simulink model "VARIACION_P1_P2_P3"  (R2019b)
settings: Solver=VariableStepAuto  StartTime=0.0  StopTime=15000  RelTol=1e-3
undefined symbols (not defined in the file): n, p1, p1Aumentado, p1Disminuido, p2, p2Aumentado, p2Disminuido, p3, p3Aumentado, p3Disminuido, p6
libraries: simulink x18
settings Model: Creator=USUARIO  LastModifiedBy=USUARIO

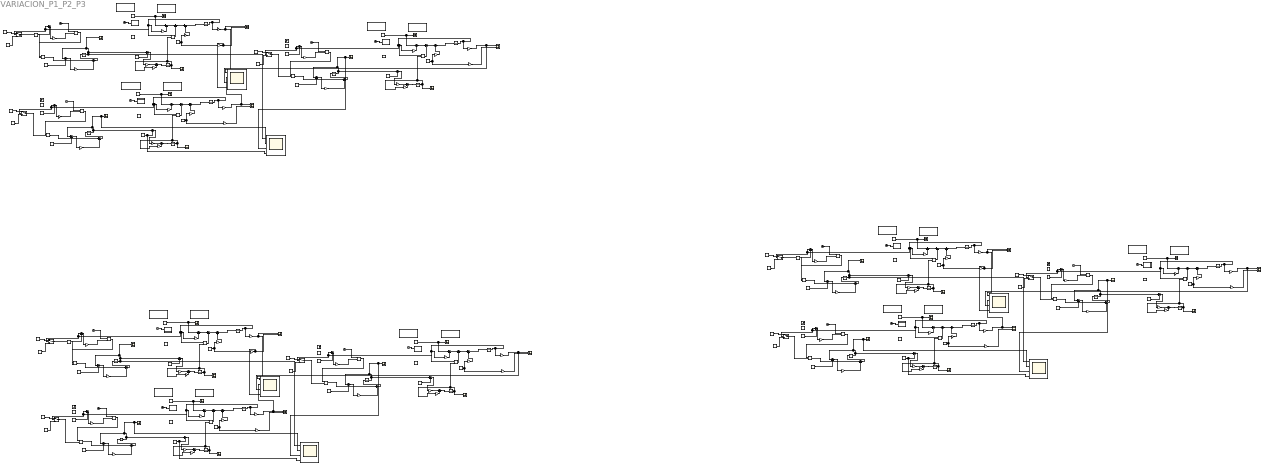
== system VARIACION_P1_P2_P3 ==
  Clock{,1..17} (18 alike) : Clock
  Constant{1..9} (9 alike) : Constant  Value=0
  Gain{1,5,11,17,19,21,23,27,32,34,37,39,41,45,50,52} (16 alike) : Gain  Gain=p1
  Gain{3..4,9..10,15..16,20,25..26,30..31,36,38,43..44,48..49,54} (18 alike) : Gain  Gain=18
  Gain{6,12,18,33,40,46,51} (7 alike) : Gain  Gain=p2
  Gain13 : Gain  Gain=p1Disminuido
  Gain{2,8,14,24,29,35,47} (7 alike) : Gain  Gain=p3
  Gain22 : Gain  Gain=p2Aumentado
  Gain28 : Gain  Gain=p2Disminuido
  Gain42 : Gain  Gain=p3Disminuido
  Gain53 : Gain  Gain=p3Aumentado
  Gain7 : Gain  Gain=p1Aumentado
  Glucosa {,1..5} (6 alike) : Constant  Value=7
  Glucosa basal{1..2,5,10..11,14,19..20,23} (9 alike) : Constant  Value=4.5
  Glucosa basal{3,6..7,12,15..16,21,24..25} (9 alike) : Constant
  Glucosa basal{4,8..9,13,17..18,22,26..27} (9 alike) : Constant  Value=0
  Grafica ingesta D{1..9} (9 alike) : Scope
  INSULINA{,1..8} (9 alike) : Scope
  Ib{,1..8} (9 alike) : Constant  Value=12
  Ingesta 75 g1 : MATLAB Function  TreatAsAtomicUnit=on
  Ingesta 75 g2 : MATLAB Function  TreatAsAtomicUnit=on
  Ingesta 75 g3 : MATLAB Function  TreatAsAtomicUnit=on
  Ingesta 75 g4 : MATLAB Function  TreatAsAtomicUnit=on
  Ingesta 75 g5 : MATLAB Function  TreatAsAtomicUnit=on
  Ingesta 75 g6 : MATLAB Function  TreatAsAtomicUnit=on
  Ingesta 75 g7 : MATLAB Function  TreatAsAtomicUnit=on
  Ingesta 75 g8 : MATLAB Function  TreatAsAtomicUnit=on
  Ingesta 75 g9 : MATLAB Function  TreatAsAtomicUnit=on
  Insulina basal{1..9} (9 alike) : Constant  Value=12
  Integrator{1,3,6,9,12,16,19,22,25} (9 alike) : Integrator  InitialCondition=7.5
  Integrator{4,7,10,13..14,17,20,23,26} (9 alike) : Integrator  InitialCondition=12
  Integrator{2,5,8,11,15,18,21,24,27} (9 alike) : Integrator
  Model Info1 : simulink/Model-Wide Utilities/Model Info  Frame=on  DisplayStringWithTags=|  HorizontalTextAlignment=Center  LeftAlignmentValue=0.5
      | Insulina constante 
      | igual a la basal
      | 
      | I(0) = Ib
  Model Info10 : simulink/Model-Wide Utilities/Model Info  Frame=on  DisplayStringWithTags=|  HorizontalTextAlignment=Center  LeftAlignmentValue=0.5
      | MODELO ORIGINAL
      | 
      | 
      | PERSONA NO DIABETICA
      | 
      | CON INSULINA VARIABLE
  Model Info11 : simulink/Model-Wide Utilities/Model Info  Frame=on  DisplayStringWithTags=|  HorizontalTextAlignment=Center  LeftAlignmentValue=0.5
      | Insulina constante 
      | igual a la basal
      | 
      | I(0) = Ib
  Model Info12 : simulink/Model-Wide Utilities/Model Info  Frame=on  DisplayStringWithTags=|  HorizontalTextAlignment=Center  LeftAlignmentValue=0.5
      | MODELO ORIGINAL
      | 
      | 
      | PERSONA NO DIABETICA
      | 
      | CON INSULINA VARIABLE
  Model Info13 : simulink/Model-Wide Utilities/Model Info  Frame=on  DisplayStringWithTags=|  HorizontalTextAlignment=Center  LeftAlignmentValue=0.5
      | Insulina constante 
      | igual a la basal
      | 
      | I(0) = Ib
  Model Info14 : simulink/Model-Wide Utilities/Model Info  Frame=on  DisplayStringWithTags=|  HorizontalTextAlignment=Center  LeftAlignmentValue=0.5
      | MODELO ORIGINAL
      | 
      | 
      | PERSONA NO DIABETICA
      | 
      | CON INSULINA VARIABLE
  Model Info15 : simulink/Model-Wide Utilities/Model Info  Frame=on  DisplayStringWithTags=|  HorizontalTextAlignment=Center  LeftAlignmentValue=0.5
      | Insulina constante 
      | igual a la basal
      | 
      | I(0) = Ib
  Model Info16 : simulink/Model-Wide Utilities/Model Info  Frame=on  DisplayStringWithTags=|  HorizontalTextAlignment=Center  LeftAlignmentValue=0.5
      | MODELO ORIGINAL
      | 
      | 
      | PERSONA NO DIABETICA
      | 
      | CON INSULINA VARIABLE
  Model Info17 : simulink/Model-Wide Utilities/Model Info  Frame=on  DisplayStringWithTags=|  HorizontalTextAlignment=Center  LeftAlignmentValue=0.5
      | Insulina constante 
      | igual a la basal
      | 
      | I(0) = Ib
  Model Info18 : simulink/Model-Wide Utilities/Model Info  Frame=on  DisplayStringWithTags=|  HorizontalTextAlignment=Center  LeftAlignmentValue=0.5
      | MODELO ORIGINAL
      | 
      | 
      | PERSONA NO DIABETICA
      | 
      | CON INSULINA VARIABLE
  Model Info2 : simulink/Model-Wide Utilities/Model Info  Frame=on  DisplayStringWithTags=|  HorizontalTextAlignment=Center  LeftAlignmentValue=0.5
      | MODELO ORIGINAL
      | 
      | 
      | PERSONA NO DIABETICA
      | 
      | CON INSULINA VARIABLE
  Model Info3 : simulink/Model-Wide Utilities/Model Info  Frame=on  DisplayStringWithTags=|  HorizontalTextAlignment=Center  LeftAlignmentValue=0.5
      | Insulina constante 
      | igual a la basal
      | 
      | I(0) = Ib
  Model Info4 : simulink/Model-Wide Utilities/Model Info  Frame=on  DisplayStringWithTags=|  HorizontalTextAlignment=Center  LeftAlignmentValue=0.5
      | MODELO ORIGINAL
      | 
      | 
      | PERSONA NO DIABETICA
      | 
      | CON INSULINA VARIABLE
  Model Info5 : simulink/Model-Wide Utilities/Model Info  Frame=on  DisplayStringWithTags=|  HorizontalTextAlignment=Center  LeftAlignmentValue=0.5
      | Insulina constante 
      | igual a la basal
      | 
      | I(0) = Ib
  Model Info6 : simulink/Model-Wide Utilities/Model Info  Frame=on  DisplayStringWithTags=|  HorizontalTextAlignment=Center  LeftAlignmentValue=0.5
      | MODELO ORIGINAL
      | 
      | 
      | PERSONA NO DIABETICA
      | 
      | CON INSULINA VARIABLE
  Model Info7 : simulink/Model-Wide Utilities/Model Info  Frame=on  DisplayStringWithTags=|  HorizontalTextAlignment=Center  LeftAlignmentValue=0.5
      | Insulina constante 
      | igual a la basal
      | 
      | I(0) = Ib
  Model Info8 : simulink/Model-Wide Utilities/Model Info  Frame=on  DisplayStringWithTags=|  HorizontalTextAlignment=Center  LeftAlignmentValue=0.5
      | MODELO ORIGINAL
      | 
      | 
      | PERSONA NO DIABETICA
      | 
      | CON INSULINA VARIABLE
  Model Info9 : simulink/Model-Wide Utilities/Model Info  Frame=on  DisplayStringWithTags=|  HorizontalTextAlignment=Center  LeftAlignmentValue=0.5
      | Insulina constante 
      | igual a la basal
      | 
      | I(0) = Ib
  Product{1..27} (27 alike) : Product
  Step{,1..5} (6 alike) : Step  Time=10  Before=7  After=4  SampleTime=0
  Sum{1..2,4..7,9..15,17..28,30..38,40..46,48..55,57..62,64..70,72} (63 alike) : Sum  Inputs=|+-
  Sum{3,8,16,29,39,47,56,63,71} (9 alike) : Sum  Inputs=|++
  Switch{,1..8} (9 alike) : Switch  Criteria=u2 > Threshold  Threshold=5
  i(T){1..9} (9 alike) : Constant  Value=12
  insulina activa{1..9} (9 alike) : Scope
  mODELO ORIGINAL{1..9} (9 alike) : Scope  NumInputPorts=2
  p{1,3,5,7,9,11,13,15,17} (9 alike) : Constant  Value=5
  p{2,4,6,8,10,12,14,16,18} (9 alike) : Gain  Gain=p6
  p4 = n{,1..8} (9 alike) : Gain  Gain=n
  variacion p1: glucosa : Scope  NumInputPorts=4
  variacion p1: glucosa1 : Scope  NumInputPorts=4
  variacion p1: glucosa2 : Scope  NumInputPorts=4
  variacion p1: insulina : Scope  NumInputPorts=4
  variacion p1: insulina1 : Scope  NumInputPorts=4
  variacion p1: insulina2 : Scope  NumInputPorts=4
  wires:
  Glucosa basal1/1 -> Gain5/1, Gain4/1  "glucosa basal"
  Gain3/1 -> variacion p1: glucosa/1, mODELO ORIGINAL1/1  "Glucosa p1 original"
  Glucosa basal7/1 -> Switch/1  "glucosa basal"
  Clock1/1 -> Ingesta 75 g1/1(in)
  p6/1 -> Product7/2
  p4/1 -> Product6/2
  p4 = n2/1 -> Sum19/2
  Integrator8/1 -> insulina activa3/1, Product5/2, Gain18/1  "X(t)"
  Sum5/1 -> Sum3/1
  p5/1 -> Sum31/2  "glucosa basal"
  Sum1/1 -> Gain2/1
  Integrator1/1 -> Gain3/1, Sum31/1, Switch/2, Product1/1, Gain1/1  "G(t)"
  Switch/1 -> Product8/2
  Gain5/1 -> Sum3/2
  Constant1/1 -> Grafica ingesta D1/1, Sum2/1
  Product1/1 -> Sum5/2
  Sum2/1 -> Sum5/1
  Gain6/1 -> Sum4/2
  Gain1/1 -> Sum2/2
  Glucosa basal8/1 -> Switch/3  "glucosa basal"
  Insulina basal1/1 -> Sum1/2  "insulina basal"
  Clock3/1 -> Ingesta 75 g2/1(in)
  Sum12/1 -> Integrator5/1
  Glucosa basal3/1 -> Switch1/1  "glucosa basal"
  Sum11/1 -> Integrator4/1
  Gain9/1 -> variacion p1: glucosa/2, mODELO ORIGINAL2/1  "Glucosa p1 aumentado"
  Product6/1 -> Product9/1
  Clock5/1 -> Ingesta 75 g3/1(in)
  Sum20/1 -> Integrator8/1
  Glucosa basal6/1 -> Switch2/1  "glucosa basal"
  Sum19/1 -> Integrator7/1
  Sum4/1 -> Integrator2/1
  Glucosa basal5/1 -> Gain17/1, Gain16/1  "glucosa basal"
  Integrator6/1 -> Gain15/1, Sum17/1, Switch2/2, Product5/1, Gain13/1  "G(t)"
  Gain14/1 -> Sum20/1
  Sum32/1 -> p4 = n/1
  Sum14/1 -> Gain14/1
  Ib1/1 -> Sum10/2  "glucosa basal"
  Gain12/1 -> Sum12/2
  Gain7/1 -> Sum7/2
  p2/1 -> Product3/2
  Clock/1 -> Product7/1
  Integrator5/1 -> insulina activa2/1, Product2/2, Gain12/1  "X(t)"
  Product4/1 -> Sum11/1
  Gain10/1 -> mODELO ORIGINAL2/2  "glucosa basal"
  Sum8/1 -> Integrator3/1
  Glucosa basal4/1 -> Switch1/3  "glucosa basal"
  Product3/1 -> Product4/1
  Clock2/1 -> Product3/1
  p3/1 -> Sum17/2  "glucosa basal"
  Glucosa basal2/1 -> Gain11/1, Gain10/1  "glucosa basal"
  Integrator4/1 -> Sum6/1, variacion p1: insulina/2, INSULINA1/1, Sum10/1  "Insulina p1 aumentado"
  Switch1/1 -> Product4/2
  Sum10/1 -> p4 = n1/1
  Gain11/1 -> Sum8/2
  Constant2/1 -> Grafica ingesta D2/1, Sum7/1
  Gain13/1 -> Sum15/2
  Ib2/1 -> Sum18/2  "glucosa basal"
  Insulina basal3/1 -> Sum14/2  "insulina basal"
  Product9/1 -> Sum19/1
  Sum16/1 -> Integrator6/1
  p4 = n1/1 -> Sum11/2
  Product2/1 -> Sum13/2
  Integrator7/1 -> Sum14/1, variacion p1: insulina/3, INSULINA2/1, Sum18/1  "Insulina p1 disminuido"
  Switch2/1 -> Product9/2
  Sum7/1 -> Sum13/1
  Product5/1 -> Sum21/2
  Product7/1 -> Product8/1
  Constant3/1 -> Grafica ingesta D3/1, Sum15/1
  Sum18/1 -> p4 = n2/1
  Sum33/1 -> Integrator14/1
  Product8/1 -> Sum33/1
  Gain4/1 -> variacion p1: glucosa/4, mODELO ORIGINAL1/2  "glucosa basal"
  Sum3/1 -> Integrator1/1
  Sum31/1 -> p6/1
  Integrator14/1 -> variacion p1: insulina/1, INSULINA/1, Sum32/1, Sum1/1  "Insulina p1 original"
  Sum17/1 -> p4/1
  Sum21/1 -> Sum16/1
  Integrator2/1 -> insulina activa1/1, Product1/2, Gain6/1  "X(t)"
  Gain17/1 -> Sum16/2
  Gain16/1 -> mODELO ORIGINAL3/2  "glucosa basal"
  Insulina basal2/1 -> variacion p1: insulina/4, Sum6/2  "insulina basal"
  Gain2/1 -> Sum4/1
  p4 = n/1 -> Sum33/2
  p1/1 -> Sum9/2  "glucosa basal"
  Sum9/1 -> p2/1
  Gain8/1 -> Sum12/1
  Gain18/1 -> Sum20/2
  Integrator3/1 -> Gain9/1, Sum9/1, Switch1/2, Product2/1, Gain7/1  "G(t)"
  Glucosa basal9/1 -> Switch2/3  "glucosa basal"
  Sum15/1 -> Sum21/1
  Sum13/1 -> Sum8/1
  Sum6/1 -> Gain8/1
  Gain15/1 -> variacion p1: glucosa/3, mODELO ORIGINAL3/1  "Glucosa p1 disminuido"
  Clock4/1 -> Product6/1
  Ib/1 -> Sum32/2  "glucosa basal"
  Sum23/1 -> p4 = n4/1
  Sum38/1 -> Sum29/1
  Insulina basal6/1 -> Sum27/2  "insulina basal"
  p11/1 -> Sum40/2  "glucosa basal"
  Sum24/1 -> Integrator13/1
  Ib3/1 -> Sum41/2  "glucosa basal"
  Switch4/1 -> Product13/2
  Sum40/1 -> p12/1
  Glucosa basal18/1 -> Switch5/3  "glucosa basal"
  p12/1 -> Product16/2
  Product16/1 -> Product17/1
  Gain25/1 -> variacion p1: glucosa2/3, mODELO ORIGINAL6/1  "Glucosa p2 disminuido"
  Clock10/1 -> Product15/1
  Clock9/1 -> Ingesta 75 g5/1(in)
  Sum43/1 -> Integrator11/1
  Sum28/1 -> Sum38/1
  Gain30/1 -> variacion p1: glucosa2/1, mODELO ORIGINAL4/1  "GGlucosa p2 original"
  Gain28/1 -> Sum37/2
  Sum45/1 -> Gain35/1
  Gain32/1 -> Sum39/2
  Integrator12/1 -> Gain36/1, Sum48/1, Switch4/2, Product11/1, Gain34/1  "G(t)"
  Insulina basal5/1 -> variacion p1: insulina2/4, Sum45/2  "insulina basal"
  Glucosa basal13/1 -> Switch4/3  "glucosa basal"
  Sum39/1 -> Integrator9/1
  Ib5/1 -> Sum34/2  "glucosa basal"
  Gain29/1 -> Sum43/1
  Gain26/1 -> mODELO ORIGINAL6/2  "glucosa basal"
  Glucosa basal10/1 -> Gain32/1, Gain31/1  "glucosa basal"
  p7/1 -> Sum48/2  "glucosa basal"
  Gain35/1 -> Sum25/1
  Constant5/1 -> Grafica ingesta D5/1, Sum46/1
  Gain27/1 -> Sum29/2
  Integrator13/1 -> Sum45/1, variacion p1: insulina2/2, INSULINA4/1, Sum23/1  "Insulina p2 aumentado"
  Product11/1 -> Sum26/2
  Sum27/1 -> Gain24/1
  Sum48/1 -> p8/1
  Gain23/1 -> Sum28/2
  Integrator10/1 -> variacion p1: insulina2/1, INSULINA3/1, Sum41/1, Sum22/1  "Insulina p2 original"
  Integrator11/1 -> insulina activa4/1, Product10/2, Gain33/1  "X(t)"
  Gain22/1 -> Sum25/2
  p8/1 -> Product12/2
  Integrator9/1 -> Gain30/1, Sum40/1, Switch3/2, Product10/1, Gain19/1  "G(t)"
  Sum41/1 -> p4 = n3/1
  Sum30/1 -> p10/1
  Product14/1 -> Sum38/2
  Glucosa basal14/1 -> Gain27/1, Gain26/1  "glucosa basal"
  Constant6/1 -> Grafica ingesta D6/1, Sum28/1
  Sum34/1 -> p4 = n5/1
  Gain34/1 -> Sum46/2
  Gain19/1 -> Sum36/2
  Sum42/1 -> Integrator10/1
  Gain36/1 -> variacion p1: glucosa2/2, mODELO ORIGINAL5/1  "Glucosa p2 aumentado"
  Product13/1 -> Sum24/1
  Product17/1 -> Sum42/1
  p9/1 -> Sum30/2  "glucosa basal"
  Glucosa basal12/1 -> Switch4/1  "glucosa basal"
  Integrator15/1 -> insulina activa5/1, Product11/2, Gain22/1  "X(t)"
  Product18/1 -> Sum35/1
  Gain31/1 -> variacion p1: glucosa2/4, mODELO ORIGINAL4/2  "glucosa basal"
  Sum37/1 -> Integrator18/1
  Integrator18/1 -> insulina activa6/1, Product14/2, Gain28/1  "X(t)"
  Gain21/1 -> Sum47/2
  Sum47/1 -> Integrator12/1
  Switch5/1 -> Product18/2
  p4 = n3/1 -> Sum42/2
  Constant4/1 -> Grafica ingesta D4/1, Sum36/1
  Glucosa basal15/1 -> Switch5/1  "glucosa basal"
  Sum46/1 -> Sum26/1
  Sum26/1 -> Sum47/1
  Sum29/1 -> Integrator16/1
  Integrator17/1 -> Sum27/1, variacion p1: insulina2/3, INSULINA5/1, Sum34/1  "Insulina p2 disminuido"
  Integrator16/1 -> Gain25/1, Sum30/1, Switch5/2, Product14/1, Gain23/1  "G(t)"
  Clock11/1 -> Ingesta 75 g6/1(in)
  Product15/1 -> Product18/1
  Glucosa basal11/1 -> Gain21/1, Gain20/1  "glucosa basal"
  Gain24/1 -> Sum37/1
  Ib4/1 -> Sum23/2  "glucosa basal"
  Sum35/1 -> Integrator17/1
  p4 = n4/1 -> Sum24/2
  Clock8/1 -> Product12/1
  Sum25/1 -> Integrator15/1
  Glucosa basal16/1 -> Switch3/1  "glucosa basal"
  Gain20/1 -> mODELO ORIGINAL5/2  "glucosa basal"
  Glucosa basal17/1 -> Switch3/3  "glucosa basal"
  Insulina basal4/1 -> Sum22/2  "insulina basal"
  Clock6/1 -> Product16/1
  Gain33/1 -> Sum43/2
  Switch3/1 -> Product17/2
  Product10/1 -> Sum44/2
  Sum44/1 -> Sum39/1
  p10/1 -> Product15/2
  p4 = n5/1 -> Sum35/2
  Product12/1 -> Product13/1
  Clock7/1 -> Ingesta 75 g4/1(in)
  Sum22/1 -> Gain29/1
  Sum36/1 -> Sum44/1
  Sum50/1 -> p4 = n7/1
  Sum62/1 -> Sum56/1
  Insulina basal9/1 -> Sum54/2  "insulina basal"
  p17/1 -> Sum64/2  "glucosa basal"
  Sum51/1 -> Integrator23/1
  Ib6/1 -> Sum65/2  "glucosa basal"
  Switch7/1 -> Product22/2
  Sum64/1 -> p18/1
  Glucosa basal27/1 -> Switch8/3  "glucosa basal"
  p18/1 -> Product25/2
  Product25/1 -> Product26/1
  Gain43/1 -> variacion p1: glucosa1/3, mODELO ORIGINAL9/1  "Glucosa p3 disminuido"
  Clock16/1 -> Product24/1
  Clock15/1 -> Ingesta 75 g8/1(in)
  Sum67/1 -> Integrator21/1
  Sum55/1 -> Sum62/1
  Gain48/1 -> variacion p1: glucosa1/1, mODELO ORIGINAL7/1  "Glucosa p3 original"
  Gain46/1 -> Sum61/2
  Sum69/1 -> Gain53/1
  Gain50/1 -> Sum63/2
  Integrator22/1 -> Gain54/1, Sum72/1, Switch7/2, Product20/1, Gain52/1  "G(t)"
  Insulina basal8/1 -> variacion p1: insulina1/4, Sum69/2  "insulina basal"
  Glucosa basal22/1 -> Switch7/3  "glucosa basal"
  Sum63/1 -> Integrator19/1
  Ib8/1 -> Sum58/2  "glucosa basal"
  Gain47/1 -> Sum67/1
  Gain44/1 -> mODELO ORIGINAL9/2  "glucosa basal"
  Glucosa basal19/1 -> Gain50/1, Gain49/1  "glucosa basal"
  p13/1 -> Sum72/2  "glucosa basal"
  Gain53/1 -> Sum52/1
  Constant8/1 -> Grafica ingesta D8/1, Sum70/1
  Gain45/1 -> Sum56/2
  Integrator23/1 -> Sum69/1, variacion p1: insulina1/2, INSULINA7/1, Sum50/1  "Insulina p3 aumentado"
  Product20/1 -> Sum53/2
  Sum54/1 -> Gain42/1
  Sum72/1 -> p14/1
  Gain41/1 -> Sum55/2
  Integrator20/1 -> variacion p1: insulina1/1, INSULINA6/1, Sum65/1, Sum49/1  "Insulina p3 original"
  Integrator21/1 -> insulina activa7/1, Product19/2, Gain51/1  "X(t)"
  Gain40/1 -> Sum52/2
  p14/1 -> Product21/2
  Integrator19/1 -> Gain48/1, Sum64/1, Switch6/2, Product19/1, Gain37/1  "G(t)"
  Sum65/1 -> p4 = n6/1
  Sum57/1 -> p16/1
  Product23/1 -> Sum62/2
  Glucosa basal23/1 -> Gain45/1, Gain44/1  "glucosa basal"
  Constant9/1 -> Grafica ingesta D9/1, Sum55/1
  Sum58/1 -> p4 = n8/1
  Gain52/1 -> Sum70/2
  Gain37/1 -> Sum60/2
  Sum66/1 -> Integrator20/1
  Gain54/1 -> variacion p1: glucosa1/2, mODELO ORIGINAL8/1  "Glucosa p3 aumentado"
  Product22/1 -> Sum51/1
  Product26/1 -> Sum66/1
  p15/1 -> Sum57/2  "glucosa basal"
  Glucosa basal21/1 -> Switch7/1  "glucosa basal"
  Integrator24/1 -> insulina activa8/1, Product20/2, Gain40/1  "X(t)"
  Product27/1 -> Sum59/1
  Gain49/1 -> variacion p1: glucosa1/4, mODELO ORIGINAL7/2  "glucosa basal"
  Sum61/1 -> Integrator27/1
  Integrator27/1 -> insulina activa9/1, Product23/2, Gain46/1  "X(t)"
  Gain39/1 -> Sum71/2
  Sum71/1 -> Integrator22/1
  Switch8/1 -> Product27/2
  p4 = n6/1 -> Sum66/2
  Constant7/1 -> Grafica ingesta D7/1, Sum60/1
  Glucosa basal24/1 -> Switch8/1  "glucosa basal"
  Sum70/1 -> Sum53/1
  Sum53/1 -> Sum71/1
  Sum56/1 -> Integrator25/1
  Integrator26/1 -> Sum54/1, variacion p1: insulina1/3, INSULINA8/1, Sum58/1  "Insulina p3 disminuido"
  Integrator25/1 -> Gain43/1, Sum57/1, Switch8/2, Product23/1, Gain41/1  "G(t)"
  Clock17/1 -> Ingesta 75 g9/1(in)
  Product24/1 -> Product27/1
  Glucosa basal20/1 -> Gain39/1, Gain38/1  "glucosa basal"
  Gain42/1 -> Sum61/1
  Ib7/1 -> Sum50/2  "glucosa basal"
  Sum59/1 -> Integrator26/1
  p4 = n7/1 -> Sum51/2
  Clock14/1 -> Product21/1
  Sum52/1 -> Integrator24/1
  Glucosa basal25/1 -> Switch6/1  "glucosa basal"
  Gain38/1 -> mODELO ORIGINAL8/2  "glucosa basal"
  Glucosa basal26/1 -> Switch6/3  "glucosa basal"
  Insulina basal7/1 -> Sum49/2  "insulina basal"
  Clock12/1 -> Product25/1
  Gain51/1 -> Sum67/2
  Switch6/1 -> Product26/2
  Product19/1 -> Sum68/2
  Sum68/1 -> Sum63/1
  p16/1 -> Product24/2
  p4 = n8/1 -> Sum59/2
  Product21/1 -> Product22/1
  Clock13/1 -> Ingesta 75 g7/1(in)
  Sum49/1 -> Gain47/1
  Sum60/1 -> Sum68/1

== matlab function VARIACION_P1_P2_P3/Ingesta 75 g1 ==
  data: in input; D output
function D = comida(in)
% Variables de entrada en la funcion
t = in(1) %- 8*60*60; % Ajuste para iniciar a las 8 de la mañana
 
% Parámetros del modelo
Ag = 0.8; % adimensional
Tmaxi = 55*60; % s
Vg = 13.79; % L
Tmaxg = 40*60; % s
t1 = 0;
Dg = 0;
f = 1000/180; % factor de conversión de g a mmol
 
% Comidas (perturbaciones) a lo largo de un día
if t >= 0 && t < 180*60 % ingesta de 75 g de HC
    t1 = 0;
    Dg = 50*f;
end
 
% Ecuación
D = (Dg*Ag*(t-t1)*exp(-(t-t1)/Tmaxi))/(Vg*Tmaxg^2);

== matlab function VARIACION_P1_P2_P3/Ingesta 75 g2 ==
  data: in input; D output
function D = comida(in)
% Variables de entrada en la funcion
t = in(1) %- 8*60*60; % Ajuste para iniciar a las 8 de la mañana
 
% Parámetros del modelo
Ag = 0.8; % adimensional
Tmaxi = 55*60; % s
Vg = 13.79; % L
Tmaxg = 40*60; % s
t1 = 0;
Dg = 0;
f = 1000/180; % factor de conversión de g a mmol
 
% Comidas (perturbaciones) a lo largo de un día
if t >= 0 && t < 180*60 % ingesta de 75 g de HC
    t1 = 0;
    Dg = 50*f;
end
 
% Ecuación
D = (Dg*Ag*(t-t1)*exp(-(t-t1)/Tmaxi))/(Vg*Tmaxg^2);

== matlab function VARIACION_P1_P2_P3/Ingesta 75 g3 ==
  data: in input; D output
function D = comida(in)
% Variables de entrada en la funcion
t = in(1) %- 8*60*60; % Ajuste para iniciar a las 8 de la mañana
 
% Parámetros del modelo
Ag = 0.8; % adimensional
Tmaxi = 55*60; % s
Vg = 13.79; % L
Tmaxg = 40*60; % s
t1 = 0;
Dg = 0;
f = 1000/180; % factor de conversión de g a mmol
 
% Comidas (perturbaciones) a lo largo de un día
if t >= 0 && t < 180*60 % ingesta de 75 g de HC
    t1 = 0;
    Dg = 50*f;
end
 
% Ecuación
D = (Dg*Ag*(t-t1)*exp(-(t-t1)/Tmaxi))/(Vg*Tmaxg^2);

== matlab function VARIACION_P1_P2_P3/Ingesta 75 g4 ==
  data: in input; D output
function D = comida(in)
% Variables de entrada en la funcion
t = in(1) %- 8*60*60; % Ajuste para iniciar a las 8 de la mañana
 
% Parámetros del modelo
Ag = 0.8; % adimensional
Tmaxi = 55*60; % s
Vg = 13.79; % L
Tmaxg = 40*60; % s
t1 = 0;
Dg = 0;
f = 1000/180; % factor de conversión de g a mmol
 
% Comidas (perturbaciones) a lo largo de un día
if t >= 0 && t < 180*60 % ingesta de 75 g de HC
    t1 = 0;
    Dg = 50*f;
end
 
% Ecuación
D = (Dg*Ag*(t-t1)*exp(-(t-t1)/Tmaxi))/(Vg*Tmaxg^2);

== matlab function VARIACION_P1_P2_P3/Ingesta 75 g5 ==
  data: in input; D output
function D = comida(in)
% Variables de entrada en la funcion
t = in(1) %- 8*60*60; % Ajuste para iniciar a las 8 de la mañana
 
% Parámetros del modelo
Ag = 0.8; % adimensional
Tmaxi = 55*60; % s
Vg = 13.79; % L
Tmaxg = 40*60; % s
t1 = 0;
Dg = 0;
f = 1000/180; % factor de conversión de g a mmol
 
% Comidas (perturbaciones) a lo largo de un día
if t >= 0 && t < 180*60 % ingesta de 75 g de HC
    t1 = 0;
    Dg = 50*f;
end
 
% Ecuación
D = (Dg*Ag*(t-t1)*exp(-(t-t1)/Tmaxi))/(Vg*Tmaxg^2);

== matlab function VARIACION_P1_P2_P3/Ingesta 75 g6 ==
  data: in input; D output
function D = comida(in)
% Variables de entrada en la funcion
t = in(1) %- 8*60*60; % Ajuste para iniciar a las 8 de la mañana
 
% Parámetros del modelo
Ag = 0.8; % adimensional
Tmaxi = 55*60; % s
Vg = 13.79; % L
Tmaxg = 40*60; % s
t1 = 0;
Dg = 0;
f = 1000/180; % factor de conversión de g a mmol
 
% Comidas (perturbaciones) a lo largo de un día
if t >= 0 && t < 180*60 % ingesta de 75 g de HC
    t1 = 0;
    Dg = 50*f;
end
 
% Ecuación
D = (Dg*Ag*(t-t1)*exp(-(t-t1)/Tmaxi))/(Vg*Tmaxg^2);

== matlab function VARIACION_P1_P2_P3/Ingesta 75 g7 ==
  data: in input; D output
function D = comida(in)
% Variables de entrada en la funcion
t = in(1) %- 8*60*60; % Ajuste para iniciar a las 8 de la mañana
 
% Parámetros del modelo
Ag = 0.8; % adimensional
Tmaxi = 55*60; % s
Vg = 13.79; % L
Tmaxg = 40*60; % s
t1 = 0;
Dg = 0;
f = 1000/180; % factor de conversión de g a mmol
 
% Comidas (perturbaciones) a lo largo de un día
if t >= 0 && t < 180*60 % ingesta de 75 g de HC
    t1 = 0;
    Dg = 50*f;
end
 
% Ecuación
D = (Dg*Ag*(t-t1)*exp(-(t-t1)/Tmaxi))/(Vg*Tmaxg^2);

== matlab function VARIACION_P1_P2_P3/Ingesta 75 g8 ==
  data: in input; D output
function D = comida(in)
% Variables de entrada en la funcion
t = in(1) %- 8*60*60; % Ajuste para iniciar a las 8 de la mañana
 
% Parámetros del modelo
Ag = 0.8; % adimensional
Tmaxi = 55*60; % s
Vg = 13.79; % L
Tmaxg = 40*60; % s
t1 = 0;
Dg = 0;
f = 1000/180; % factor de conversión de g a mmol
 
% Comidas (perturbaciones) a lo largo de un día
if t >= 0 && t < 180*60 % ingesta de 75 g de HC
    t1 = 0;
    Dg = 50*f;
end
 
% Ecuación
D = (Dg*Ag*(t-t1)*exp(-(t-t1)/Tmaxi))/(Vg*Tmaxg^2);

== matlab function VARIACION_P1_P2_P3/Ingesta 75 g9 ==
  data: in input; D output
function D = comida(in)
% Variables de entrada en la funcion
t = in(1) %- 8*60*60; % Ajuste para iniciar a las 8 de la mañana
 
% Parámetros del modelo
Ag = 0.8; % adimensional
Tmaxi = 55*60; % s
Vg = 13.79; % L
Tmaxg = 40*60; % s
t1 = 0;
Dg = 0;
f = 1000/180; % factor de conversión de g a mmol
 
% Comidas (perturbaciones) a lo largo de un día
if t >= 0 && t < 180*60 % ingesta de 75 g de HC
    t1 = 0;
    Dg = 50*f;
end
 
% Ecuación
D = (Dg*Ag*(t-t1)*exp(-(t-t1)/Tmaxi))/(Vg*Tmaxg^2);
